simulink model "problem1"  (R2020b)
settings: Solver=FixedStepDiscrete  StartTime=0.0  StopTime=100  RelTol=1e-3
settings Model: Creator=Nitin  LastModifiedBy=Nitin

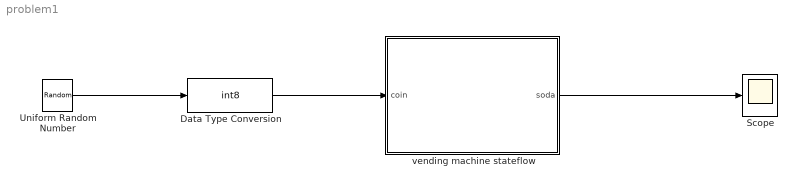
== system problem1 ==
  Data Type Conversion : DataTypeConversion  OutDataTypeStr=int8  RndMeth=Nearest
  Scope : Scope
  Uniform Random Number : UniformRandomNumber  Minimum=0  Maximum=2  Seed=330  SampleTime=10
  vending machine stateflow : Stateflow chart  TreatAsAtomicUnit=on
  wires:
  Uniform Random Number/1 -> Data Type Conversion/1
  vending machine stateflow/1(soda) -> Scope/1
  Data Type Conversion/1 -> vending machine stateflow/1(coin)

== stateflow chart problem1/vending machine stateflow ==
  state got_nothing
  state got_nickel
  state got_dime
  (default) -> got_nothing
  got_nothing -> got_nickel [order 1] : [coin==1]{soda=0}
  got_nickel -> got_nothing [order 1] : [coin==2]{soda=1}
  got_nothing -> got_dime [order 2] : [coin==2]{soda=0}
  got_dime -> got_nothing [order 2] : [coin==1]{soda=1}
  got_nickel -> got_dime [order 2] : [coin==1]{soda=0}
  got_dime -> got_nickel [order 1] : [coin==2]{soda=1}
  data: coin input; soda output
